simulink model "test_mdl_NI"  (R2018a)
settings: Solver=VariableStepAuto  StartTime=0.0  StopTime=10.0  RelTol=1e-3
(part 23 of 24)

== system test_mdl_NI/CAN_Signal/GWM/Other_GWMTx/CruiseCtrl_Strg_Data_FD1/CcAslButtnSetDecPress2 ==
  in : Inport
  out : Outport
  wires:
  in/1 -> out/1

== system test_mdl_NI/CAN_Signal/GWM/Other_GWMTx/CruiseCtrl_Strg_Data_FD1/CcAslButtnSetIncPress2 ==
  in : Inport
  out : Outport
  wires:
  in/1 -> out/1

== system test_mdl_NI/CAN_Signal/GWM/Other_GWMTx/CruiseCtrl_Strg_Data_FD1/CcAslButtnSetPress2 ==
  in : Inport
  out : Outport
  wires:
  in/1 -> out/1

== system test_mdl_NI/CAN_Signal/GWM/Other_GWMTx/CruiseCtrl_Strg_Data_FD1/CcAsllButtnResPress2 ==
  in : Inport
  out : Outport
  wires:
  in/1 -> out/1

== system test_mdl_NI/CAN_Signal/GWM/Other_GWMTx/CruiseCtrl_Strg_Data_FD1/CcButtnOffPress2 ==
  in : Inport
  out : Outport
  wires:
  in/1 -> out/1

== system test_mdl_NI/CAN_Signal/GWM/Other_GWMTx/CruiseCtrl_Strg_Data_FD1/CcButtnOnOffCnclPress2 ==
  in : Inport
  out : Outport
  wires:
  in/1 -> out/1

== system test_mdl_NI/CAN_Signal/GWM/Other_GWMTx/CruiseCtrl_Strg_Data_FD1/CcButtnOnOffPress2 ==
  in : Inport
  out : Outport
  wires:
  in/1 -> out/1

== system test_mdl_NI/CAN_Signal/GWM/Other_GWMTx/CruiseCtrl_Strg_Data_FD1/CcButtnOnPress2 ==
  in : Inport
  out : Outport
  wires:
  in/1 -> out/1

== system test_mdl_NI/CAN_Signal/GWM/Other_GWMTx/CruiseCtrl_Strg_Data_FD1/SelDrvMdeAdptSte_D_Stat ==
  in : Inport
  out : Outport
  wires:
  in/1 -> out/1

== system test_mdl_NI/CAN_Signal/GWM/Other_GWMTx/CruiseCtrl_Strg_Data_FD1/TjaButtnOnOffPress2 ==
  in : Inport
  out : Outport
  wires:
  in/1 -> out/1

== system test_mdl_NI/CAN_Signal/GWM/Other_GWMTx/DCACA_Data1_FD1/CoolFanDcac_D_Rq ==
  in : Inport
  out : Outport
  wires:
  in/1 -> out/1

== system test_mdl_NI/CAN_Signal/GWM/Other_GWMTx/DCACA_Data1_FD1/DcacClntFlw_D_Rq ==
  in : Inport
  out : Outport
  wires:
  in/1 -> out/1

== system test_mdl_NI/CAN_Signal/GWM/Other_GWMTx/DCACA_Data1_FD1/DcacPlugPrsnt_B_Stat ==
  in : Inport
  out : Outport
  wires:
  in/1 -> out/1

== system test_mdl_NI/CAN_Signal/GWM/Other_GWMTx/DCACA_Data1_FD1/DcacRdy_D_Stat ==
  in : Inport
  out : Outport
  wires:
  in/1 -> out/1

== system test_mdl_NI/CAN_Signal/GWM/Other_GWMTx/DCACA_Data2_FD1/DcacIn_I_Actl ==
  in : Inport
  out : Outport
  wires:
  in/1 -> out/1

== system test_mdl_NI/CAN_Signal/GWM/Other_GWMTx/DCACA_Data2_FD1/DcacIn_U_Actl ==
  in : Inport
  out : Outport
  wires:
  in/1 -> out/1

== system test_mdl_NI/CAN_Signal/GWM/Other_GWMTx/DCACA_Data2_FD1/Dcac_Te_Actl ==
  in : Inport
  out : Outport
  wires:
  in/1 -> out/1

== system test_mdl_NI/CAN_Signal/GWM/Other_GWMTx/DCACA_Data3_FD1/DcacIn_Pw_Mx ==
  in : Inport
  out : Outport
  wires:
  in/1 -> out/1

== system test_mdl_NI/CAN_Signal/GWM/Other_GWMTx/DCACA_Data3_FD1/DcacOut1_Pw_Actl ==
  in : Inport
  out : Outport
  wires:
  in/1 -> out/1

== system test_mdl_NI/CAN_Signal/GWM/Other_GWMTx/DCACA_Data3_FD1/DcacOut2_Pw_Actl ==
  in : Inport
  out : Outport
  wires:
  in/1 -> out/1

== system test_mdl_NI/CAN_Signal/GWM/Other_GWMTx/DCACA_Data3_FD1/DcacOut_Pw_Mx ==
  in : Inport
  out : Outport
  wires:
  in/1 -> out/1

== system test_mdl_NI/CAN_Signal/GWM/Other_GWMTx/DifferentialCtrlData_1_FD1/RearDiffLck_Tq_Actl2 ==
  in : Inport
  out : Outport
  wires:
  in/1 -> out/1

== system test_mdl_NI/CAN_Signal/GWM/Other_GWMTx/Driver_Dr_Stat_FD1/BLISLEDStatDriverSide ==
  in : Inport
  out : Outport
  wires:
  in/1 -> out/1

== system test_mdl_NI/CAN_Signal/GWM/Other_GWMTx/Driver_Dr_Stat_FD1/ChildLckFdbckRd_B_Stat ==
  in : Inport
  out : Outport
  wires:
  in/1 -> out/1

== system test_mdl_NI/CAN_Signal/GWM/Other_GWMTx/Driver_Dr_Stat_FD1/ChildLckPw_D_Rq ==
  in : Inport
  out : Outport
  wires:
  in/1 -> out/1

== system test_mdl_NI/CAN_Signal/GWM/Other_GWMTx/Driver_Dr_Stat_FD1/ChildLckPw_N_Cnt ==
  in : Inport
  out : Outport
  wires:
  in/1 -> out/1

== system test_mdl_NI/CAN_Signal/GWM/Other_GWMTx/Driver_Dr_Stat_FD1/Driver_Lock_Sw_Cnt ==
  in : Inport
  out : Outport
  wires:
  in/1 -> out/1

== system test_mdl_NI/CAN_Signal/GWM/Other_GWMTx/Driver_Dr_Stat_FD1/Driver_Lock_Sw_Stat ==
  in : Inport
  out : Outport
  wires:
  in/1 -> out/1

== system test_mdl_NI/CAN_Signal/GWM/Other_GWMTx/Driver_Dr_Stat_FD1/KeyCylSwDrvDr_D_Stat ==
  in : Inport
  out : Outport
  wires:
  in/1 -> out/1

== system test_mdl_NI/CAN_Signal/GWM/Other_GWMTx/Driver_Dr_Stat_FD1/RollCodeDrvDrKeyCyl ==
  in : Inport
  out : Outport
  wires:
  in/1 -> out/1

== system test_mdl_NI/CAN_Signal/GWM/Other_GWMTx/Driver_Dr_Stat_FD1/RvrseMirrorChime_B_Rq ==
  in : Inport
  out : Outport
  wires:
  in/1 -> out/1

== system test_mdl_NI/CAN_Signal/GWM/Other_GWMTx/Driver_Dr_Stat_FD1/WndwDrvSide_D_Stat ==
  in : Inport
  out : Outport
  wires:
  in/1 -> out/1

== system test_mdl_NI/CAN_Signal/GWM/Other_GWMTx/Dsp_Request_Signals11_FD1/ApaMdeStat_D_RqDrv ==
  in : Inport
  out : Outport
  wires:
  in/1 -> out/1

== system test_mdl_NI/CAN_Signal/GWM/Other_GWMTx/Dsp_Request_Signals11_FD1/ApaSwtch_D_RqMnu ==
  in : Inport
  out : Outport
  wires:
  in/1 -> out/1

== system test_mdl_NI/CAN_Signal/GWM/Other_GWMTx/Dsp_Request_Signals11_FD1/CamAutoTowbarZoom ==
  in : Inport
  out : Outport
  wires:
  in/1 -> out/1

== system test_mdl_NI/CAN_Signal/GWM/Other_GWMTx/Dsp_Request_Signals11_FD1/CamraOvrlDyn_D_Rq ==
  in : Inport
  out : Outport
  wires:
  in/1 -> out/1

== system test_mdl_NI/CAN_Signal/GWM/Other_GWMTx/Dsp_Request_Signals11_FD1/CamraOvrlStat_D_Rq ==
  in : Inport
  out : Outport
  wires:
  in/1 -> out/1

== system test_mdl_NI/CAN_Signal/GWM/Other_GWMTx/Dsp_Request_Signals11_FD1/CamraViewSplit_B_Rq ==
  in : Inport
  out : Outport
  wires:
  in/1 -> out/1

== system test_mdl_NI/CAN_Signal/GWM/Other_GWMTx/Dsp_Request_Signals11_FD1/CamraZoomMan_D_Rq ==
  in : Inport
  out : Outport
  wires:
  in/1 -> out/1

== system test_mdl_NI/CAN_Signal/GWM/Other_GWMTx/Dsp_Request_Signals11_FD1/DistanceBarSetting ==
  in : Inport
  out : Outport
  wires:
  in/1 -> out/1

== system test_mdl_NI/CAN_Signal/GWM/Other_GWMTx/Dsp_Request_Signals11_FD1/PrkAidSwtch_D_RqMnu ==
  in : Inport
  out : Outport
  wires:
  in/1 -> out/1

== system test_mdl_NI/CAN_Signal/GWM/Other_GWMTx/ElecHorizon_Data1_FD1/EhData1_No_Actl ==
  in : Inport
  out : Outport
  wires:
  in/1 -> out/1

== system test_mdl_NI/CAN_Signal/GWM/Other_GWMTx/ElecHorizon_Data2_FD1/EhData2_No_Actl ==
  in : Inport
  out : Outport
  wires:
  in/1 -> out/1

== system test_mdl_NI/CAN_Signal/GWM/Other_GWMTx/FourByFourSwitchData_FD1/AwdLck_D_RqDrv ==
  in : Inport
  out : Outport
  wires:
  in/1 -> out/1

== system test_mdl_NI/CAN_Signal/GWM/Other_GWMTx/FourByFourSwitchData_FD1/AwdMde_D_RqDrv ==
  in : Inport
  out : Outport
  wires:
  in/1 -> out/1

== system test_mdl_NI/CAN_Signal/GWM/Other_GWMTx/FourByFourSwitchData_FD1/DrvSlipCtlMde_B_Rq3 ==
  in : Inport
  out : Outport
  wires:
  in/1 -> out/1

== system test_mdl_NI/CAN_Signal/GWM/Other_GWMTx/FourByFourSwitchData_FD1/HdcSwtchPos_B_Actl ==
  in : Inport
  out : Outport
  wires:
  in/1 -> out/1

== system test_mdl_NI/CAN_Signal/GWM/Other_GWMTx/FourByFourSwitchData_FD1/HybMdeSwtch_B_Rq ==
  in : Inport
  out : Outport
  wires:
  in/1 -> out/1

== system test_mdl_NI/CAN_Signal/GWM/Other_GWMTx/FourByFourSwitchData_FD1/RearDiffLck_D_RqDrv ==
  in : Inport
  out : Outport
  wires:
  in/1 -> out/1

== system test_mdl_NI/CAN_Signal/GWM/Other_GWMTx/FourByFourSwitchData_FD1/TrailCtlSwtch_B_Stat3 ==
  in : Inport
  out : Outport
  wires:
  in/1 -> out/1

== system test_mdl_NI/CAN_Signal/GWM/Other_GWMTx/Front_Distance_Req_FD1/FdsmTrgCntr_B_Actl ==
  in : Inport
  out : Outport
  wires:
  in/1 -> out/1

== system test_mdl_NI/CAN_Signal/GWM/Other_GWMTx/Front_Distance_Req_FD1/FdsmTrgDist_L_Actl ==
  in : Inport
  out : Outport
  wires:
  in/1 -> out/1

== system test_mdl_NI/CAN_Signal/GWM/Other_GWMTx/Front_Distance_Req_FD1/FdsmTrgLeft_B_Actl ==
  in : Inport
  out : Outport
  wires:
  in/1 -> out/1

== system test_mdl_NI/CAN_Signal/GWM/Other_GWMTx/Front_Distance_Req_FD1/FdsmTrgRight_B_Actl ==
  in : Inport
  out : Outport
  wires:
  in/1 -> out/1

== system test_mdl_NI/CAN_Signal/GWM/Other_GWMTx/Front_Distance_Req_FD1/LscmbbBaSens_D_Rq ==
  in : Inport
  out : Outport
  wires:
  in/1 -> out/1

== system test_mdl_NI/CAN_Signal/GWM/Other_GWMTx/Front_Distance_Req_FD1/LscmbbBlck_B_Actl ==
  in : Inport
  out : Outport
  wires:
  in/1 -> out/1

== system test_mdl_NI/CAN_Signal/GWM/Other_GWMTx/Front_Distance_Req_FD1/LscmbbBrkDecel_A_Rq ==
  in : Inport
  out : Outport
  wires:
  in/1 -> out/1

== system test_mdl_NI/CAN_Signal/GWM/Other_GWMTx/Front_Distance_Req_FD1/LscmbbBrkDecel_B_Enbl ==
  in : Inport
  out : Outport
  wires:
  in/1 -> out/1

== system test_mdl_NI/CAN_Signal/GWM/Other_GWMTx/Front_Distance_Req_FD1/LscmbbBrkDecel_No_Cnt ==
  in : Inport
  out : Outport
  wires:
  in/1 -> out/1

== system test_mdl_NI/CAN_Signal/GWM/Other_GWMTx/Front_Distance_Req_FD1/LscmbbBrkDecel_No_Cs ==
  in : Inport
  out : Outport
  wires:
  in/1 -> out/1

== system test_mdl_NI/CAN_Signal/GWM/Other_GWMTx/Front_Distance_Req_FD1/LscmbbBrkPrchg_D_Rq ==
  in : Inport
  out : Outport
  wires:
  in/1 -> out/1

== system test_mdl_NI/CAN_Signal/GWM/Other_GWMTx/Front_Distance_Req_FD1/LscmbbDeny_B_Actl ==
  in : Inport
  out : Outport
  wires:
  in/1 -> out/1

== system test_mdl_NI/CAN_Signal/GWM/Other_GWMTx/Front_Distance_Req_FD1/LscmbbEngTqMn_B_Rq ==
  in : Inport
  out : Outport
  wires:
  in/1 -> out/1

== system test_mdl_NI/CAN_Signal/GWM/Other_GWMTx/Front_Distance_Req_FD1/LscmbbMsgTxt_D_Rq ==
  in : Inport
  out : Outport
  wires:
  in/1 -> out/1

== system test_mdl_NI/CAN_Signal/GWM/Other_GWMTx/Front_Distance_Req_FD1/LscmbbPostEvnt_B_Dsply ==
  in : Inport
  out : Outport
  wires:
  in/1 -> out/1

== system test_mdl_NI/CAN_Signal/GWM/Other_GWMTx/Front_Distance_Req_FD1/LscmbbSrvcRqd_B_Rq ==
  in : Inport
  out : Outport
  wires:
  in/1 -> out/1

== system test_mdl_NI/CAN_Signal/GWM/Other_GWMTx/Front_Distance_Req_FD1/WndwFrontHeat_B_Rq ==
  in : Inport
  out : Outport
  wires:
  in/1 -> out/1

== system test_mdl_NI/CAN_Signal/GWM/Other_GWMTx/GGCC_Config_Mgmt_ID_1_FD1/VehicleGGCCData ==
  in : Inport
  out : Outport
  wires:
  in/1 -> out/1

== system test_mdl_NI/CAN_Signal/GWM/Other_GWMTx/GWM_AutoSar_NetMgmt_FD1/GWM_AutoSarNMControl ==
  in : Inport
  out : Outport
  wires:
  in/1 -> out/1

== system test_mdl_NI/CAN_Signal/GWM/Other_GWMTx/GWM_AutoSar_NetMgmt_FD1/GWM_AutoSarNMNodeId ==
  in : Inport
  out : Outport
  wires:
  in/1 -> out/1

== system test_mdl_NI/CAN_Signal/GWM/Other_GWMTx/GWM_AutoSar_NetMgmt_FD1/GWM_AutoSarNMReserved1 ==
  in : Inport
  out : Outport
  wires:
  in/1 -> out/1

== system test_mdl_NI/CAN_Signal/GWM/Other_GWMTx/GWM_AutoSar_NetMgmt_FD1/GWM_AutoSarNMReserved2 ==
  in : Inport
  out : Outport
  wires:
  in/1 -> out/1

== system test_mdl_NI/CAN_Signal/GWM/Other_GWMTx/GWM_AutoSar_NetMgmt_FD1/GWM_AutoSarNMReserved3 ==
  in : Inport
  out : Outport
  wires:
  in/1 -> out/1

== system test_mdl_NI/CAN_Signal/GWM/Other_GWMTx/GWM_AutoSar_NetMgmt_FD1/GWM_AutoSarNMReserved4 ==
  in : Inport
  out : Outport
  wires:
  in/1 -> out/1

== system test_mdl_NI/CAN_Signal/GWM/Other_GWMTx/GWM_AutoSar_NetMgmt_FD1/GWM_GWNMProxy ==
  in : Inport
  out : Outport
  wires:
  in/1 -> out/1

== system test_mdl_NI/CAN_Signal/GWM/Other_GWMTx/GWM_AutoSar_NetMgmt_FD1/GWM_GWOnBoardTester ==
  in : Inport
  out : Outport
  wires:
  in/1 -> out/1

== system test_mdl_NI/CAN_Signal/GWM/Other_GWMTx/GlobalClock_Data_FD1/GlblClkDay_No_Actl ==
  in : Inport
  out : Outport
  wires:
  in/1 -> out/1

== system test_mdl_NI/CAN_Signal/GWM/Other_GWMTx/GlobalClock_Data_FD1/GlblClkHr_No_Actl ==
  in : Inport
  out : Outport
  wires:
  in/1 -> out/1

== system test_mdl_NI/CAN_Signal/GWM/Other_GWMTx/GlobalClock_Data_FD1/GlblClkMnte_No_Actl ==
  in : Inport
  out : Outport
  wires:
  in/1 -> out/1

== system test_mdl_NI/CAN_Signal/GWM/Other_GWMTx/GlobalClock_Data_FD1/GlblClkScnd_No_Actl ==
  in : Inport
  out : Outport
  wires:
  in/1 -> out/1

== system test_mdl_NI/CAN_Signal/GWM/Other_GWMTx/GlobalClock_Data_FD1/GlblClkYr_No_Actl ==
  in : Inport
  out : Outport
  wires:
  in/1 -> out/1

== system test_mdl_NI/CAN_Signal/GWM/Other_GWMTx/Global_PATS_Cntrl_Info_FD1/immoControlCmd_T1 ==
  in : Inport
  out : Outport
  wires:
  in/1 -> out/1

== system test_mdl_NI/CAN_Signal/GWM/Other_GWMTx/Global_PATS_Cntrl_Info_FD1/immoControlData_T1 ==
  in : Inport
  out : Outport
  wires:
  in/1 -> out/1

== system test_mdl_NI/CAN_Signal/GWM/Other_GWMTx/IPC_Infotainment_FD1/BeltminderAudioMute ==
  in : Inport
  out : Outport
  wires:
  in/1 -> out/1

== system test_mdl_NI/CAN_Signal/GWM/Other_GWMTx/IPC_Infotainment_FD1/Chime_Source ==
  in : Inport
  out : Outport
  wires:
  in/1 -> out/1

== system test_mdl_NI/CAN_Signal/GWM/Other_GWMTx/IPC_Infotainment_FD1/HdcOn_B_Rq ==
  in : Inport
  out : Outport
  wires:
  in/1 -> out/1

== system test_mdl_NI/CAN_Signal/GWM/Other_GWMTx/IPC_Infotainment_FD1/IPC_Attn_Info_Audio ==
  in : Inport
  out : Outport
  wires:
  in/1 -> out/1

== system test_mdl_NI/CAN_Signal/GWM/Other_GWMTx/IPC_Infotainment_FD1/IPC_MyKeyVolLimit_St ==
  in : Inport
  out : Outport
  wires:
  in/1 -> out/1

== system test_mdl_NI/CAN_Signal/GWM/Other_GWMTx/IPC_Infotainment_FD1/IPC_New_Attn_Event ==
  in : Inport
  out : Outport
  wires:
  in/1 -> out/1

== system test_mdl_NI/CAN_Signal/GWM/Other_GWMTx/IPC_Infotainment_FD1/Power_Up_Chime_Modules ==
  in : Inport
  out : Outport
  wires:
  in/1 -> out/1

== system test_mdl_NI/CAN_Signal/GWM/Other_GWMTx/IPC_Infotainment_FD1/Veh_V2_Dsply ==
  in : Inport
  out : Outport
  wires:
  in/1 -> out/1

== system test_mdl_NI/CAN_Signal/GWM/Other_GWMTx/IPC_Send_Signals_2_FD1/ElLongTerm_L_Dsply ==
  in : Inport
  out : Outport
  wires:
  in/1 -> out/1

== system test_mdl_NI/CAN_Signal/GWM/Other_GWMTx/IPC_Send_Signals_2_FD1/ElTrip_L_Dsply ==
  in : Inport
  out : Outport
  wires:
  in/1 -> out/1

== system test_mdl_NI/CAN_Signal/GWM/Other_GWMTx/IPC_Send_Signals_2_FD1/FuelRange_L_Dsply ==
  in : Inport
  out : Outport
  wires:
  in/1 -> out/1

== system test_mdl_NI/CAN_Signal/GWM/Other_GWMTx/MHT_EV_Wakeup_FD1/BattChlrSov_B_Rq ==
  in : Inport
  out : Outport
  wires:
  in/1 -> out/1

== system test_mdl_NI/CAN_Signal/GWM/Other_GWMTx/MHT_EV_Wakeup_FD1/BattChrgTrgtSoC_D_Rq ==
  in : Inport
  out : Outport
  wires:
  in/1 -> out/1

== system test_mdl_NI/CAN_Signal/GWM/Other_GWMTx/MHT_EV_Wakeup_FD1/BattTracDrvSustn_B_Rq ==
  in : Inport
  out : Outport
  wires:
  in/1 -> out/1

== system test_mdl_NI/CAN_Signal/GWM/Other_GWMTx/MHT_EV_Wakeup_FD1/BrkAppl_D_RqPt ==
  in : Inport
  out : Outport
  wires:
  in/1 -> out/1

== system test_mdl_NI/CAN_Signal/GWM/Other_GWMTx/MHT_EV_Wakeup_FD1/CabnEvapSovFront_B_Rq ==
  in : Inport
  out : Outport
  wires:
  in/1 -> out/1

== system test_mdl_NI/CAN_Signal/GWM/Other_GWMTx/MHT_EV_Wakeup_FD1/CabnEvapSovRear_B_Rq ==
  in : Inport
  out : Outport
  wires:
  in/1 -> out/1

== system test_mdl_NI/CAN_Signal/GWM/Other_GWMTx/MHT_EV_Wakeup_FD1/HeatCoreSovRear_B_Rq ==
  in : Inport
  out : Outport
  wires:
  in/1 -> out/1

== system test_mdl_NI/CAN_Signal/GWM/Other_GWMTx/MHT_EV_Wakeup_FD1/HtrnClntFlw_D_Rq ==
  in : Inport
  out : Outport
  wires:
  in/1 -> out/1

== system test_mdl_NI/CAN_Signal/GWM/Other_GWMTx/MHT_EV_Wakeup_FD1/HtrnCnnctPwr_B_Stat ==
  in : Inport
  out : Outport
  wires:
  in/1 -> out/1

== system test_mdl_NI/CAN_Signal/GWM/Other_GWMTx/MHT_EV_Wakeup_FD1/HtrnDcdcDis_B_Rq ==
  in : Inport
  out : Outport
  wires:
  in/1 -> out/1

== system test_mdl_NI/CAN_Signal/GWM/Other_GWMTx/MHT_EV_Wakeup_FD1/PtcHtr_D_Stat ==
  in : Inport
  out : Outport
  wires:
  in/1 -> out/1

== system test_mdl_NI/CAN_Signal/GWM/Other_GWMTx/Mc_Send_Signals_2_FD1/BttOn_B_Rq ==
  in : Inport
  out : Outport
  wires:
  in/1 -> out/1

== system test_mdl_NI/CAN_Signal/GWM/Other_GWMTx/Mc_Send_Signals_2_FD1/Btt_L_Actl ==
  in : Inport
  out : Outport
  wires:
  in/1 -> out/1

== system test_mdl_NI/CAN_Signal/GWM/Other_GWMTx/Mc_Send_Signals_2_FD1/EngExhMdeQuiet_D_Rq ==
  in : Inport
  out : Outport
  wires:
  in/1 -> out/1

== system test_mdl_NI/CAN_Signal/GWM/Other_GWMTx/Mc_Send_Signals_2_FD1/EsaOn_B_Rq ==
  in : Inport
  out : Outport
  wires:
  in/1 -> out/1

== system test_mdl_NI/CAN_Signal/GWM/Other_GWMTx/Mc_Send_Signals_2_FD1/Mc_VehLangUsrSel_St ==
  in : Inport
  out : Outport
  wires:
  in/1 -> out/1

== system test_mdl_NI/CAN_Signal/GWM/Other_GWMTx/Mc_Send_Signals_2_FD1/Mc_VehUnitTempUsrSel_St ==
  in : Inport
  out : Outport
  wires:
  in/1 -> out/1

== system test_mdl_NI/CAN_Signal/GWM/Other_GWMTx/Mc_Send_Signals_2_FD1/Mc_VehUntTrpCoUsrSel_St ==
  in : Inport
  out : Outport
  wires:
  in/1 -> out/1

== system test_mdl_NI/CAN_Signal/GWM/Other_GWMTx/Mc_Send_Signals_2_FD1/SelDrvMdeDsply_B_Avail ==
  in : Inport
  out : Outport
  wires:
  in/1 -> out/1

== system test_mdl_NI/CAN_Signal/GWM/Other_GWMTx/Mc_Send_Signals_2_FD1/SelDrvMdeTxtReset_B_Rq ==
  in : Inport
  out : Outport
  wires:
  in/1 -> out/1

== system test_mdl_NI/CAN_Signal/GWM/Other_GWMTx/Mc_Send_Signals_2_FD1/WaitToStartLamp_D_Falt ==
  in : Inport
  out : Outport
  wires:
  in/1 -> out/1

== system test_mdl_NI/CAN_Signal/GWM/Other_GWMTx/ParkAid_Aud_Warn_CmdM_FD1/Cta_D_Rq ==
  in : Inport
  out : Outport
  wires:
  in/1 -> out/1

== system test_mdl_NI/CAN_Signal/GWM/Other_GWMTx/ParkAid_Aud_Warn_CmdM_FD1/PrkAidRear_D_RqDrv ==
  in : Inport
  out : Outport
  wires:
  in/1 -> out/1

== system test_mdl_NI/CAN_Signal/GWM/Other_GWMTx/ParkAid_Aud_Warn_CmdM_FD1/Sod_D_Rq ==
  in : Inport
  out : Outport
  wires:
  in/1 -> out/1

== system test_mdl_NI/CAN_Signal/GWM/Other_GWMTx/ParkAid_Aud_Warn_CmdM_FD1/SteEffort_D_Rq ==
  in : Inport
  out : Outport
  wires:
  in/1 -> out/1

== system test_mdl_NI/CAN_Signal/GWM/Other_GWMTx/Pass_Dr_Stat_FD1/BLISLEDStatPassSide ==
  in : Inport
  out : Outport
  wires:
  in/1 -> out/1

== system test_mdl_NI/CAN_Signal/GWM/Other_GWMTx/Pass_Dr_Stat_FD1/ChildLckFdbckRp_B_Stat ==
  in : Inport
  out : Outport
  wires:
  in/1 -> out/1

== system test_mdl_NI/CAN_Signal/GWM/Other_GWMTx/Pass_Dr_Stat_FD1/Memory_1_SwPsngr_Stat ==
  in : Inport
  out : Outport
  wires:
  in/1 -> out/1

== system test_mdl_NI/CAN_Signal/GWM/Other_GWMTx/Pass_Dr_Stat_FD1/Memory_2_SwPsngr_Stat ==
  in : Inport
  out : Outport
  wires:
  in/1 -> out/1

== system test_mdl_NI/CAN_Signal/GWM/Other_GWMTx/Pass_Dr_Stat_FD1/Memory_3_SwPsngr_Stat ==
  in : Inport
  out : Outport
  wires:
  in/1 -> out/1

== system test_mdl_NI/CAN_Signal/GWM/Other_GWMTx/Pass_Dr_Stat_FD1/Pasngr_Lock_Sw_Cnt ==
  in : Inport
  out : Outport
  wires:
  in/1 -> out/1

== system test_mdl_NI/CAN_Signal/GWM/Other_GWMTx/Pass_Dr_Stat_FD1/Pasngr_Lock_Sw_Stat ==
  in : Inport
  out : Outport
  wires:
  in/1 -> out/1

== system test_mdl_NI/CAN_Signal/GWM/Other_GWMTx/Pass_Dr_Stat_FD1/RollCode_No_ActlPdm ==
  in : Inport
  out : Outport
  wires:
  in/1 -> out/1

== system test_mdl_NI/CAN_Signal/GWM/Other_GWMTx/Pass_Dr_Stat_FD1/WndwPsngrSide_D_Stat ==
  in : Inport
  out : Outport
  wires:
  in/1 -> out/1

== system test_mdl_NI/CAN_Signal/GWM/Other_GWMTx/Personality_APIM_Data_FD1/CtrStkDsplyOp_D_Rq ==
  in : Inport
  out : Outport
  wires:
  in/1 -> out/1

== system test_mdl_NI/CAN_Signal/GWM/Other_GWMTx/Personality_APIM_Data_FD1/CtrStkFeatConfigActl ==
  in : Inport
  out : Outport
  wires:
  in/1 -> out/1

== system test_mdl_NI/CAN_Signal/GWM/Other_GWMTx/Personality_APIM_Data_FD1/CtrStkFeatNoActl ==
  in : Inport
  out : Outport
  wires:
  in/1 -> out/1

== system test_mdl_NI/CAN_Signal/GWM/Other_GWMTx/Personality_APIM_Data_FD1/CtrStkPersIndex_D_Actl ==
  in : Inport
  out : Outport
  wires:
  in/1 -> out/1

== system test_mdl_NI/CAN_Signal/GWM/Other_GWMTx/Personality_APIM_Data_FD1/Pers1OptIn_B_Stats ==
  in : Inport
  out : Outport
  wires:
  in/1 -> out/1

== system test_mdl_NI/CAN_Signal/GWM/Other_GWMTx/Personality_APIM_Data_FD1/Pers2OptIn_B_Stats ==
  in : Inport
  out : Outport
  wires:
  in/1 -> out/1

== system test_mdl_NI/CAN_Signal/GWM/Other_GWMTx/Personality_APIM_Data_FD1/Pers3OptIn_B_Stats ==
  in : Inport
  out : Outport
  wires:
  in/1 -> out/1

== system test_mdl_NI/CAN_Signal/GWM/Other_GWMTx/Personality_APIM_Data_FD1/Pers4OptIn_B_Stats ==
  in : Inport
  out : Outport
  wires:
  in/1 -> out/1

== system test_mdl_NI/CAN_Signal/GWM/Other_GWMTx/Personality_APIM_Data_FD1/PersStore_D_Rq ==
  in : Inport
  out : Outport
  wires:
  in/1 -> out/1

== system test_mdl_NI/CAN_Signal/GWM/Other_GWMTx/Personality_Data_FD1/MsgCntrDsplyOp_D_Rq ==
  in : Inport
  out : Outport
  wires:
  in/1 -> out/1

== system test_mdl_NI/CAN_Signal/GWM/Other_GWMTx/Personality_Data_FD1/MsgCntrFeatConfigRq ==
  in : Inport
  out : Outport
  wires:
  in/1 -> out/1

== system test_mdl_NI/CAN_Signal/GWM/Other_GWMTx/Personality_Data_FD1/MsgCntrFeatNoRq ==
  in : Inport
  out : Outport
  wires:
  in/1 -> out/1

== system test_mdl_NI/CAN_Signal/GWM/Other_GWMTx/Personality_Data_FD1/MsgCntrPersIndex_D_Rq ==
  in : Inport
  out : Outport
  wires:
  in/1 -> out/1

== system test_mdl_NI/CAN_Signal/GWM/Other_GWMTx/Power_Liftgate_Stat_FD1/DrLckCnt_No_ActlTgate ==
  in : Inport
  out : Outport
  wires:
  in/1 -> out/1

== system test_mdl_NI/CAN_Signal/GWM/Other_GWMTx/Power_Liftgate_Stat_FD1/DrTGate_D_Rq ==
  in : Inport
  out : Outport
  wires:
  in/1 -> out/1

== system test_mdl_NI/CAN_Signal/GWM/Other_GWMTx/Power_Liftgate_Stat_FD1/DrTgateChime2_D_Rq ==
  in : Inport
  out : Outport
  wires:
  in/1 -> out/1

== system test_mdl_NI/CAN_Signal/GWM/Other_GWMTx/Power_Liftgate_Stat_FD1/Power_Liftgate_Mode_Stt ==
  in : Inport
  out : Outport
  wires:
  in/1 -> out/1

== system test_mdl_NI/CAN_Signal/GWM/Other_GWMTx/Power_Liftgate_Stat_FD1/PwLftgtIntSw_B_Stat ==
  in : Inport
  out : Outport
  wires:
  in/1 -> out/1

== system test_mdl_NI/CAN_Signal/GWM/Other_GWMTx/PreCond_Hev_Data1_FD1/ChrgStat_D2_Dsply ==
  in : Inport
  out : Outport
  wires:
  in/1 -> out/1

== system test_mdl_NI/CAN_Signal/GWM/Other_GWMTx/PreCond_Hev_Data2_FD1/BattTracClntFlw_Pc_Rq ==
  in : Inport
  out : Outport
  wires:
  in/1 -> out/1

== system test_mdl_NI/CAN_Signal/GWM/Other_GWMTx/PreCond_Hev_Data2_FD1/BattTrac_I_EstVsc ==
  in : Inport
  out : Outport
  wires:
  in/1 -> out/1

== system test_mdl_NI/CAN_Signal/GWM/Other_GWMTx/PreCond_Hev_Data2_FD1/DrvCondTpRrDefrs_B_Rq ==
  in : Inport
  out : Outport
  wires:
  in/1 -> out/1

== system test_mdl_NI/CAN_Signal/GWM/Other_GWMTx/PreCond_Hev_Data2_FD1/HtrnAin_UHi_Actl ==
  in : Inport
  out : Outport
  wires:
  in/1 -> out/1

== system test_mdl_NI/CAN_Signal/GWM/Other_GWMTx/PreCond_Hev_Data2_FD1/HtrnHvilOpen_B_Actl ==
  in : Inport
  out : Outport
  wires:
  in/1 -> out/1

== system test_mdl_NI/CAN_Signal/GWM/Other_GWMTx/PreCond_Hev_Data2_FD1/HtrnMil_D_Rq ==
  in : Inport
  out : Outport
  wires:
  in/1 -> out/1

== system test_mdl_NI/CAN_Signal/GWM/Other_GWMTx/PreCond_Hev_Data2_FD1/HtrnOvrTeLamp_B_Dsply ==
  in : Inport
  out : Outport
  wires:
  in/1 -> out/1

== system test_mdl_NI/CAN_Signal/GWM/Other_GWMTx/PreCond_Hev_Data2_FD1/HtrnSrvcRqd_B_Dsply ==
  in : Inport
  out : Outport
  wires:
  in/1 -> out/1

== system test_mdl_NI/CAN_Signal/GWM/Other_GWMTx/PreCond_Hev_Data2_FD1/PreCondActv_B_Actl ==
  in : Inport
  out : Outport
  wires:
  in/1 -> out/1

== system test_mdl_NI/CAN_Signal/GWM/Other_GWMTx/PreCond_Hev_Data2_FD1/PtWakeupDeltaT_T_Rq ==
  in : Inport
  out : Outport
  wires:
  in/1 -> out/1

== system test_mdl_NI/CAN_Signal/GWM/Other_GWMTx/Suspension_Data_FD1/SuspClkSync_No_Rq ==
  in : Inport
  out : Outport
  wires:
  in/1 -> out/1

== system test_mdl_NI/CAN_Signal/GWM/Other_GWMTx/Suspension_Data_FD1/SuspFrntRight_L_Actl ==
  in : Inport
  out : Outport
  wires:
  in/1 -> out/1

== system test_mdl_NI/CAN_Signal/GWM/Other_GWMTx/Suspension_Data_FD1/SuspFrnt_L_Actl ==
  in : Inport
  out : Outport
  wires:
  in/1 -> out/1

== system test_mdl_NI/CAN_Signal/GWM/Other_GWMTx/Suspension_Data_FD1/SuspFrnt_L_Prev ==
  in : Inport
  out : Outport
  wires:
  in/1 -> out/1

== system test_mdl_NI/CAN_Signal/GWM/Other_GWMTx/Suspension_Data_FD1/SuspRearRight_L_Actl ==
  in : Inport
  out : Outport
  wires:
  in/1 -> out/1

== system test_mdl_NI/CAN_Signal/GWM/Other_GWMTx/Suspension_Data_FD1/SuspRear_L_Actl ==
  in : Inport
  out : Outport
  wires:
  in/1 -> out/1

== system test_mdl_NI/CAN_Signal/GWM/Other_GWMTx/Suspension_Data_FD1/SuspRear_L_Prev ==
  in : Inport
  out : Outport
  wires:
  in/1 -> out/1

== system test_mdl_NI/CAN_Signal/GWM/Other_GWMTx/TesterPhysicalResGWM_FD1/TesterPhysicalResGWM_F1 ==
  in : Inport
  out : Outport
  wires:
  in/1 -> out/1

== system test_mdl_NI/CAN_Signal/GWM/Other_GWMTx/TrailerAid_Data_FD1/TrlBrkInitOut_D_Rq ==
  in : Inport
  out : Outport
  wires:
  in/1 -> out/1

== system test_mdl_NI/CAN_Signal/GWM/Other_GWMTx/TrailerAid_Data_FD1/TrlrAidEnbl_D_Rq ==
  in : Inport
  out : Outport
  wires:
  in/1 -> out/1

== system test_mdl_NI/CAN_Signal/GWM/Other_GWMTx/TrailerAid_Data_FD1/TrlrAidSetup_D_Rq ==
  in : Inport
  out : Outport
  wires:
  in/1 -> out/1

== system test_mdl_NI/CAN_Signal/GWM/Other_GWMTx/TrailerAid_Data_FD1/TrlrAnOffstDir_D_Mem ==
  in : Inport
  out : Outport
  wires:
  in/1 -> out/1

== system test_mdl_NI/CAN_Signal/GWM/Other_GWMTx/TrailerAid_Data_FD1/TrlrAnOffst_An_Mem ==
  in : Inport
  out : Outport
  wires:
  in/1 -> out/1

== system test_mdl_NI/CAN_Signal/GWM/Other_GWMTx/TrailerAid_Data_FD1/TrlrAxleToBmpr_L_Actl ==
  in : Inport
  out : Outport
  wires:
  in/1 -> out/1

== system test_mdl_NI/CAN_Signal/GWM/Other_GWMTx/TrailerAid_Data_FD1/TrlrBallToBmpr_L_Actl ==
  in : Inport
  out : Outport
  wires:
  in/1 -> out/1

== system test_mdl_NI/CAN_Signal/GWM/Other_GWMTx/TrailerAid_Data_FD1/TrlrId_No_Actl ==
  in : Inport
  out : Outport
  wires:
  in/1 -> out/1

== system test_mdl_NI/CAN_Signal/GWM/Other_GWMTx/TrailerAid_Data_FD1/TrlrRvrseCancl_B_Rq ==
  in : Inport
  out : Outport
  wires:
  in/1 -> out/1

== system test_mdl_NI/CAN_Signal/GWM/Other_GWMTx/TrailerAid_Data_FD1/TrlrTrgtOffst_L_Actl ==
  in : Inport
  out : Outport
  wires:
  in/1 -> out/1

== system test_mdl_NI/CAN_Signal/GWM/Other_GWMTx/TrailerAid_Data_FD1/TrlrTrgtPtrnId_No_Mem ==
  in : Inport
  out : Outport
  wires:
  in/1 -> out/1

== system test_mdl_NI/CAN_Signal/GWM/Other_GWMTx/TrailerAid_Data_FD1/TrlrTrgtToBmpr_L_Actl ==
  in : Inport
  out : Outport
  wires:
  in/1 -> out/1

== system test_mdl_NI/CAN_Signal/GWM/Other_GWMTx/TrailerAid_Stat1_FD1/TrlrSnsId_No_Actl ==
  in : Inport
  out : Outport
  wires:
  in/1 -> out/1

== system test_mdl_NI/CAN_Signal/GWM/Other_GWMTx/TrailerAid_Stat2_FD1/TrlrHitYaw_AnRate_Actl ==
  in : Inport
  out : Outport
  wires:
  in/1 -> out/1

== system test_mdl_NI/CAN_Signal/GWM/Other_GWMTx/TrailerAid_Stat2_FD1/TrlrHitchYaw_An_Actl ==
  in : Inport
  out : Outport
  wires:
  in/1 -> out/1

== system test_mdl_NI/CAN_Signal/GWM/Other_GWMTx/TrailerAid_Stat2_FD1/TrlrHitchYaw_D_Stat ==
  in : Inport
  out : Outport
  wires:
  in/1 -> out/1

== system test_mdl_NI/CAN_Signal/GWM/Other_GWMTx/TrailerAid_Stat2_FD1/TrlrYawWActl_D_Qf ==
  in : Inport
  out : Outport
  wires:
  in/1 -> out/1

== system test_mdl_NI/CAN_Signal/GWM/Other_GWMTx/TrailerAid_Stat2_FD1/TrlrYaw_W_Actl ==
  in : Inport
  out : Outport
  wires:
  in/1 -> out/1

== system test_mdl_NI/CAN_Signal/GWM/Other_GWMTx/TrailerBrakeInfo_FD1/StopLamp_B_RqTrlrBrk ==
  in : Inport
  out : Outport
  wires:
  in/1 -> out/1

== system test_mdl_NI/CAN_Signal/GWM/Other_GWMTx/TrailerBrakeInfo_FD1/TrlBrkInitOut_D_Stat ==
  in : Inport
  out : Outport
  wires:
  in/1 -> out/1

== system test_mdl_NI/CAN_Signal/GWM/Other_GWMTx/TrailerBrakeInfo_FD1/TrlrBrkActCirct_B_Falt ==
  in : Inport
  out : Outport
  wires:
  in/1 -> out/1

== system test_mdl_NI/CAN_Signal/GWM/Other_GWMTx/TrailerBrakeInfo_FD1/TrlrBrkActCnnct_B_Actl ==
  in : Inport
  out : Outport
  wires:
  in/1 -> out/1

== system test_mdl_NI/CAN_Signal/GWM/Other_GWMTx/TrailerBrakeInfo_FD1/TrlrBrkCtl_B_Falt ==
  in : Inport
  out : Outport
  wires:
  in/1 -> out/1

== system test_mdl_NI/CAN_Signal/GWM/Other_GWMTx/TrailerBrakeInfo_FD1/TrlrBrkDcnnt_B_Actl ==
  in : Inport
  out : Outport
  wires:
  in/1 -> out/1

== system test_mdl_NI/CAN_Signal/GWM/Other_GWMTx/TrailerBrakeInfo_FD1/TrlrBrkDsply_B_Rq ==
  in : Inport
  out : Outport
  wires:
  in/1 -> out/1

== system test_mdl_NI/CAN_Signal/GWM/Other_GWMTx/TrailerBrakeInfo_FD1/TrlrBrkGain_No_Actl ==
  in : Inport
  out : Outport
  wires:
  in/1 -> out/1

== system test_mdl_NI/CAN_Signal/GWM/Other_GWMTx/TrailerBrakeInfo_FD1/TrlrBrkMde_D_Actl ==
  in : Inport
  out : Outport
  wires:
  in/1 -> out/1

== system test_mdl_NI/CAN_Signal/GWM/Other_GWMTx/TrailerBrakeInfo_FD1/TrlrBrkOut_No_Dsply ==
  in : Inport
  out : Outport
  wires:
  in/1 -> out/1

== system test_mdl_NI/CAN_Signal/GWM/Other_GWMTx/TrailerInfo_2_FD1/TrlrAidAn_URate_Actl ==
  in : Inport
  out : Outport
  wires:
  in/1 -> out/1

== system test_mdl_NI/CAN_Signal/GWM/Other_GWMTx/TrailerInfo_2_FD1/TrlrAidAn_U_Actl ==
  in : Inport
  out : Outport
  wires:
  in/1 -> out/1

== system test_mdl_NI/CAN_Signal/GWM/Other_GWMTx/TrailerInfo_2_FD1/TrlrAidCtl_U_RqDrv ==
  in : Inport
  out : Outport
  wires:
  in/1 -> out/1

== system test_mdl_NI/CAN_Signal/GWM/Other_GWMTx/TrailerInfo_2_FD1/TrlrAidSwtch_D_RqDrv ==
  in : Inport
  out : Outport
  wires:
  in/1 -> out/1

== system test_mdl_NI/CAN_Signal/GWM/Other_GWMTx/TrailerInfo_FD1/ParkLampTrlrOut_B_Stat ==
  in : Inport
  out : Outport
  wires:
  in/1 -> out/1

== system test_mdl_NI/CAN_Signal/GWM/Other_GWMTx/TrailerInfo_FD1/StopLampTrlrOut_B_Stat ==
  in : Inport
  out : Outport
  wires:
  in/1 -> out/1

== system test_mdl_NI/CAN_Signal/GWM/Other_GWMTx/TrailerInfo_FD1/TrlrBattChrg_D_Stat ==
  in : Inport
  out : Outport
  wires:
  in/1 -> out/1

== system test_mdl_NI/CAN_Signal/GWM/Other_GWMTx/TrailerInfo_FD1/TrlrLampCnnct_B_Actl ==
  in : Inport
  out : Outport
  wires:
  in/1 -> out/1

== system test_mdl_NI/CAN_Signal/GWM/Other_GWMTx/TrailerInfo_FD1/TrlrLampCtl_D_Stat ==
  in : Inport
  out : Outport
  wires:
  in/1 -> out/1

== system test_mdl_NI/CAN_Signal/GWM/Other_GWMTx/TrailerInfo_FD1/TurnLampTrlrRl_B_Stat ==
  in : Inport
  out : Outport
  wires:
  in/1 -> out/1

== system test_mdl_NI/CAN_Signal/GWM/Other_GWMTx/TrailerInfo_FD1/TurnLampTrlrRr_B_Stat ==
  in : Inport
  out : Outport
  wires:
  in/1 -> out/1

== system test_mdl_NI/CAN_Signal/GWM/Other_GWMTx/VeyDynamics_Data_FD1/AdptDrvMdeChassis_D_Rq ==
  in : Inport
  out : Outport
  wires:
  in/1 -> out/1

== system test_mdl_NI/CAN_Signal/GWM/Other_GWMTx/VeyDynamics_Data_FD1/AdptDrvMdePt_D_Rq ==
  in : Inport
  out : Outport
  wires:
  in/1 -> out/1

== system test_mdl_NI/CAN_Signal/GWM/Other_GWMTx/VeyDynamics_Data_FD1/AirSprngRateFl_D_Rq ==
  in : Inport
  out : Outport
  wires:
  in/1 -> out/1

== system test_mdl_NI/CAN_Signal/GWM/Other_GWMTx/VeyDynamics_Data_FD1/AirSprngRateFr_D_Rq ==
  in : Inport
  out : Outport
  wires:
  in/1 -> out/1

== system test_mdl_NI/CAN_Signal/GWM/Other_GWMTx/VeyDynamics_Data_FD1/AirSprngRateRl_D_Rq ==
  in : Inport
  out : Outport
  wires:
  in/1 -> out/1

== system test_mdl_NI/CAN_Signal/GWM/Other_GWMTx/VeyDynamics_Data_FD1/AirSprngRateRr_D_Rq ==
  in : Inport
  out : Outport
  wires:
  in/1 -> out/1

== system test_mdl_NI/CAN_Signal/GWM/Other_GWMTx/VeyDynamics_Data_FD1/AirSuspMsgTxt_D_Rq ==
  in : Inport
  out : Outport
  wires:
  in/1 -> out/1

== system test_mdl_NI/CAN_Signal/GWM/Other_GWMTx/VeyDynamics_Data_FD1/AirSusp_D_Stat ==
  in : Inport
  out : Outport
  wires:
  in/1 -> out/1

== system test_mdl_NI/CAN_Signal/GWM/Other_GWMTx/VeyDynamics_Data_FD1/BrkPadMsgTxt_D_Rq ==
  in : Inport
  out : Outport
  wires:
  in/1 -> out/1

== system test_mdl_NI/CAN_Signal/GWM/Other_GWMTx/VeyDynamics_Data_FD1/CcdMsgTxt_D_RqDsply ==
  in : Inport
  out : Outport
  wires:
  in/1 -> out/1

== system test_mdl_NI/CAN_Signal/GWM/Other_GWMTx/VeyDynamics_Data_FD1/Ccd_B_Falt ==
  in : Inport
  out : Outport
  wires:
  in/1 -> out/1

== system test_mdl_NI/CAN_Signal/GWM/Other_GWMTx/VeyDynamics_Data_FD1/SelDrvMdeSusp_D_Stat ==
  in : Inport
  out : Outport
  wires:
  in/1 -> out/1

== system test_mdl_NI/CAN_Signal/GWM/Other_GWMTx/VeyDynamics_Data_FD1/SuspDrvMde_D_Stat ==
  in : Inport
  out : Outport
  wires:
  in/1 -> out/1

== system test_mdl_NI/CAN_Signal/GWM/Other_GWMTx/VeyDynamics_Data_FD1/SuspType_B_Stat ==
  in : Inport
  out : Outport
  wires:
  in/1 -> out/1

== system test_mdl_NI/CAN_Signal/GWM/Other_GWMTx/VeyDynamics_Data_FD1/SuspVLim_B_Rq ==
  in : Inport
  out : Outport
  wires:
  in/1 -> out/1

== system test_mdl_NI/CAN_Signal/GWM/RCM/RCMSerialNumber_FD1_454/RCMSerialNoByte1 ==
  in : Inport
  out : Outport
  wires:
  in/1 -> out/1

== system test_mdl_NI/CAN_Signal/GWM/RCM/RCMSerialNumber_FD1_454/RCMSerialNoByte2 ==
  in : Inport
  out : Outport
  wires:
  in/1 -> out/1

== system test_mdl_NI/CAN_Signal/GWM/RCM/RCMSerialNumber_FD1_454/RCMSerialNoByte3 ==
  in : Inport
  out : Outport
  wires:
  in/1 -> out/1

== system test_mdl_NI/CAN_Signal/GWM/RCM/RCMSerialNumber_FD1_454/RCMSerialNoByte4 ==
  in : Inport
  out : Outport
  wires:
  in/1 -> out/1

== system test_mdl_NI/CAN_Signal/GWM/RCM/RCMSerialNumber_FD1_454/RCMSerialNoByte5 ==
  in : Inport
  out : Outport
  wires:
  in/1 -> out/1

== system test_mdl_NI/CAN_Signal/GWM/RCM/RCMSerialNumber_FD1_454/RCMSerialNoByte6 ==
  in : Inport
  out : Outport
  wires:
  in/1 -> out/1

== system test_mdl_NI/CAN_Signal/GWM/RCM/RCMSerialNumber_FD1_454/RCMSerialNoByte7 ==
  in : Inport
  out : Outport
  wires:
  in/1 -> out/1

== system test_mdl_NI/CAN_Signal/GWM/RCM/RCMSerialNumber_FD1_454/RCMSerialNoByte8 ==
  in : Inport
  out : Outport
  wires:
  in/1 -> out/1

== system test_mdl_NI/CAN_Signal/GWM/RCM/RCMStatusMessage2_FD1_4C/EDRTriggerEvntSync ==
  in : Inport
  out : Outport
  wires:
  in/1 -> out/1

== system test_mdl_NI/CAN_Signal/GWM/RCM/RCMStatusMessage2_FD1_4C/FirstRowBuckleDriver ==
  in : Inport
  out : Outport
  wires:
  in/1 -> out/1

== system test_mdl_NI/CAN_Signal/GWM/RCM/RCMStatusMessage2_FD1_4C/FirstRowBuckleMid ==
  in : Inport
  out : Outport
  wires:
  in/1 -> out/1

== system test_mdl_NI/CAN_Signal/GWM/RCM/RCMStatusMessage2_FD1_4C/FirstRowBucklePsngr ==
  in : Inport
  out : Outport
  wires:
  in/1 -> out/1

== system test_mdl_NI/CAN_Signal/GWM/RCM/RCMStatusMessage2_FD1_4C/PassRstrnInd_Req ==
  in : Inport
  out : Outport
  wires:
  in/1 -> out/1

== system test_mdl_NI/CAN_Signal/GWM/RCM/RCMStatusMessage2_FD1_4C/PsngrFmidDetct_D_Actl ==
  in : Inport
  out : Outport
  wires:
  in/1 -> out/1

== system test_mdl_NI/CAN_Signal/GWM/RCM/RCMStatusMessage2_FD1_4C/PsngrFrntDetct_D_Actl ==
  in : Inport
  out : Outport
  wires:
  in/1 -> out/1

== system test_mdl_NI/CAN_Signal/GWM/RCM/RCMStatusMessage2_FD1_4C/RILReq ==
  in : Inport
  out : Outport
  wires:
  in/1 -> out/1

== system test_mdl_NI/CAN_Signal/GWM/RCM/RCMStatusMessage2_FD1_4C/RstrnImpactEvntStatus ==
  in : Inport
  out : Outport
  wires:
  in/1 -> out/1

== system test_mdl_NI/CAN_Signal/GWM/RCM/RCMStatusMessage2_FD1_4C/RstrnPsngrOn_D_Stat ==
  in : Inport
  out : Outport
  wires:
  in/1 -> out/1

== system test_mdl_NI/CAN_Signal/GWM/RCM/RCMStatusMessage2_FD1_4C/SecondRowBuckleDriver ==
  in : Inport
  out : Outport
  wires:
  in/1 -> out/1

== system test_mdl_NI/CAN_Signal/GWM/RCM/RCMStatusMessage2_FD1_4C/SecondRowBuckleMid ==
  in : Inport
  out : Outport
  wires:
  in/1 -> out/1

== system test_mdl_NI/CAN_Signal/GWM/RCM/RCMStatusMessage2_FD1_4C/SecondRowBucklePsngr ==
  in : Inport
  out : Outport
  wires:
  in/1 -> out/1

== system test_mdl_NI/CAN_Signal/GWM/RCM/RCMStatusMessage2_FD1_4C/ThirdRowBuckleDriver ==
  in : Inport
  out : Outport
  wires:
  in/1 -> out/1

== system test_mdl_NI/CAN_Signal/GWM/RCM/RCMStatusMessage2_FD1_4C/ThirdRowBuckleMid ==
  in : Inport
  out : Outport
  wires:
  in/1 -> out/1

== system test_mdl_NI/CAN_Signal/GWM/RCM/RCMStatusMessage2_FD1_4C/ThirdRowBucklePsngr ==
  in : Inport
  out : Outport
  wires:
  in/1 -> out/1

== system test_mdl_NI/CAN_Signal/GWM/SCCM/Steering_Data_FD1_83/AccButtnGapDecPress ==
  in : Inport
  out : Outport
  wires:
  in/1 -> out/1

== system test_mdl_NI/CAN_Signal/GWM/SCCM/Steering_Data_FD1_83/AccButtnGapIncPress ==
  in : Inport
  out : Outport
  wires:
  in/1 -> out/1

== system test_mdl_NI/CAN_Signal/GWM/SCCM/Steering_Data_FD1_83/AccButtnGapTogglePress ==
  in : Inport
  out : Outport
  wires:
  in/1 -> out/1

== system test_mdl_NI/CAN_Signal/GWM/SCCM/Steering_Data_FD1_83/AhbStat_B_Dsply ==
  in : Inport
  out : Outport
  wires:
  in/1 -> out/1

== system test_mdl_NI/CAN_Signal/GWM/SCCM/Steering_Data_FD1_83/AslButtnOnOffCnclPress ==
  in : Inport
  out : Outport
  wires:
  in/1 -> out/1

== system test_mdl_NI/CAN_Signal/GWM/SCCM/Steering_Data_FD1_83/AslButtnOnOffPress ==
  in : Inport
  out : Outport
  wires:
  in/1 -> out/1

== system test_mdl_NI/CAN_Signal/GWM/SCCM/Steering_Data_FD1_83/CcAslButtnCnclPress ==
  in : Inport
  out : Outport
  wires:
  in/1 -> out/1

== system test_mdl_NI/CAN_Signal/GWM/SCCM/Steering_Data_FD1_83/CcAslButtnCnclResPress ==
  in : Inport
  out : Outport
  wires:
  in/1 -> out/1

== system test_mdl_NI/CAN_Signal/GWM/SCCM/Steering_Data_FD1_83/CcAslButtnDeny_B_Actl ==
  in : Inport
  out : Outport
  wires:
  in/1 -> out/1

== system test_mdl_NI/CAN_Signal/GWM/SCCM/Steering_Data_FD1_83/CcAslButtnIndxDecPress ==
  in : Inport
  out : Outport
  wires:
  in/1 -> out/1

== system test_mdl_NI/CAN_Signal/GWM/SCCM/Steering_Data_FD1_83/CcAslButtnIndxIncPress ==
  in : Inport
  out : Outport
  wires:
  in/1 -> out/1

== system test_mdl_NI/CAN_Signal/GWM/SCCM/Steering_Data_FD1_83/CcAslButtnOffCnclPress ==
  in : Inport
  out : Outport
  wires:
  in/1 -> out/1

== system test_mdl_NI/CAN_Signal/GWM/SCCM/Steering_Data_FD1_83/CcAslButtnOnOffCncl ==
  in : Inport
  out : Outport
  wires:
  in/1 -> out/1

== system test_mdl_NI/CAN_Signal/GWM/SCCM/Steering_Data_FD1_83/CcAslButtnOnPress ==
  in : Inport
  out : Outport
  wires:
  in/1 -> out/1

== system test_mdl_NI/CAN_Signal/GWM/SCCM/Steering_Data_FD1_83/CcAslButtnResDecPress ==
  in : Inport
  out : Outport
  wires:
  in/1 -> out/1

== system test_mdl_NI/CAN_Signal/GWM/SCCM/Steering_Data_FD1_83/CcAslButtnResIncPress ==
  in : Inport
  out : Outport
  wires:
  in/1 -> out/1

== system test_mdl_NI/CAN_Signal/GWM/SCCM/Steering_Data_FD1_83/CcAslButtnSetDecPress ==
  in : Inport
  out : Outport
  wires:
  in/1 -> out/1

== system test_mdl_NI/CAN_Signal/GWM/SCCM/Steering_Data_FD1_83/CcAslButtnSetIncPress ==
  in : Inport
  out : Outport
  wires:
  in/1 -> out/1

== system test_mdl_NI/CAN_Signal/GWM/SCCM/Steering_Data_FD1_83/CcAslButtnSetPress ==
  in : Inport
  out : Outport
  wires:
  in/1 -> out/1

== system test_mdl_NI/CAN_Signal/GWM/SCCM/Steering_Data_FD1_83/CcAsllButtnResPress ==
  in : Inport
  out : Outport
  wires:
  in/1 -> out/1

== system test_mdl_NI/CAN_Signal/GWM/SCCM/Steering_Data_FD1_83/CcButtnOffPress ==
  in : Inport
  out : Outport
  wires:
  in/1 -> out/1

== system test_mdl_NI/CAN_Signal/GWM/SCCM/Steering_Data_FD1_83/CcButtnOnOffCnclPress ==
  in : Inport
  out : Outport
  wires:
  in/1 -> out/1

== system test_mdl_NI/CAN_Signal/GWM/SCCM/Steering_Data_FD1_83/CcButtnOnOffPress ==
  in : Inport
  out : Outport
  wires:
  in/1 -> out/1

== system test_mdl_NI/CAN_Signal/GWM/SCCM/Steering_Data_FD1_83/CcButtnOnPress ==
  in : Inport
  out : Outport
  wires:
  in/1 -> out/1

== system test_mdl_NI/CAN_Signal/GWM/SCCM/Steering_Data_FD1_83/HeadLghtHiCtrl_D_RqAhb ==
  in : Inport
  out : Outport
  wires:
  in/1 -> out/1

== system test_mdl_NI/CAN_Signal/GWM/SCCM/Steering_Data_FD1_83/HeadLghtHiFlash_D_Actl ==
  in : Inport
  out : Outport
  wires:
  in/1 -> out/1

== system test_mdl_NI/CAN_Signal/GWM/SCCM/Steering_Data_FD1_83/HeadLghtHiFlash_D_Stat ==
  in : Inport
  out : Outport
  wires:
  in/1 -> out/1

== system test_mdl_NI/CAN_Signal/GWM/SCCM/Steering_Data_FD1_83/HeadLghtHiOn_B_StatAhb ==
  in : Inport
  out : Outport
  wires:
  in/1 -> out/1

== system test_mdl_NI/CAN_Signal/GWM/SCCM/Steering_Data_FD1_83/LaSwtchPos_D_Stat ==
  in : Inport
  out : Outport
  wires:
  in/1 -> out/1

== system test_mdl_NI/CAN_Signal/GWM/SCCM/Steering_Data_FD1_83/LghtAmb_D_Sns ==
  in : Inport
  out : Outport
  wires:
  in/1 -> out/1

== system test_mdl_NI/CAN_Signal/GWM/SCCM/Steering_Data_FD1_83/TjaButtnOnOffPress ==
  in : Inport
  out : Outport
  wires:
  in/1 -> out/1

== system test_mdl_NI/CAN_Signal/GWM/SCCM/Steering_Data_FD1_83/TurnLghtSwtch_D_Stat ==
  in : Inport
  out : Outport
  wires:
  in/1 -> out/1

== system test_mdl_NI/CAN_Signal/GWM/SCCM/Steering_Data_FD1_83/WiprFrontSwtch_D_Stat ==
  in : Inport
  out : Outport
  wires:
  in/1 -> out/1

== system test_mdl_NI/CAN_Signal/GWM/SCCM/Steering_Data_FD1_83/WiprFront_D_Stat ==
  in : Inport
  out : Outport
  wires:
  in/1 -> out/1

== system test_mdl_NI/CAN_Signal/GWM/SCCM/Steering_Wheel_Data2_FD1_81/SelDrvMdeDec_B_RqDrv ==
  in : Inport
  out : Outport
  wires:
  in/1 -> out/1

== system test_mdl_NI/CAN_Signal/GWM/SCCM/Steering_Wheel_Data2_FD1_81/SelDrvMdeInc_B_RqDrv ==
  in : Inport
  out : Outport
  wires:
  in/1 -> out/1

== system test_mdl_NI/CAN_Signal/GWM/SCCM/Steering_Wheel_Data2_FD1_81/SelDrvMdeSwtch_D_Stat4 ==
  in : Inport
  out : Outport
  wires:
  in/1 -> out/1

== system test_mdl_NI/CAN_Signal/GWM/SCCM/Steering_Wheel_Data2_FD1_81/SteEffortInc_B_RqDrv ==
  in : Inport
  out : Outport
  wires:
  in/1 -> out/1

== system test_mdl_NI/CAN_Signal/GWM/SCCM/Steering_Wheel_Data2_FD1_81/SteWhlSwtchBack_B_Stat ==
  in : Inport
  out : Outport
  wires:
  in/1 -> out/1

== system test_mdl_NI/CAN_Signal/GWM/SCCM/Steering_Wheel_Data2_FD1_81/SteWhlSwtchDown_B_Stat ==
  in : Inport
  out : Outport
  wires:
  in/1 -> out/1

== system test_mdl_NI/CAN_Signal/GWM/SCCM/Steering_Wheel_Data2_FD1_81/SteWhlSwtchHome_B_Stat ==
  in : Inport
  out : Outport
  wires:
  in/1 -> out/1

== system test_mdl_NI/CAN_Signal/GWM/SCCM/Steering_Wheel_Data2_FD1_81/SteWhlSwtchHud_B_Stat ==
  in : Inport
  out : Outport
  wires:
  in/1 -> out/1

== system test_mdl_NI/CAN_Signal/GWM/SCCM/Steering_Wheel_Data2_FD1_81/SteWhlSwtchInfo_B_Stat ==
  in : Inport
  out : Outport
  wires:
  in/1 -> out/1

== system test_mdl_NI/CAN_Signal/GWM/SCCM/Steering_Wheel_Data2_FD1_81/SteWhlSwtchIod_B_Stat ==
  in : Inport
  out : Outport
  wires:
  in/1 -> out/1

== system test_mdl_NI/CAN_Signal/GWM/SCCM/Steering_Wheel_Data2_FD1_81/SteWhlSwtchLeft_B_Stat ==
  in : Inport
  out : Outport
  wires:
  in/1 -> out/1

== system test_mdl_NI/CAN_Signal/GWM/SCCM/Steering_Wheel_Data2_FD1_81/SteWhlSwtchMed_B_Stat ==
  in : Inport
  out : Outport
  wires:
  in/1 -> out/1

== system test_mdl_NI/CAN_Signal/GWM/SCCM/Steering_Wheel_Data2_FD1_81/SteWhlSwtchMenu_B_Stat ==
  in : Inport
  out : Outport
  wires:
  in/1 -> out/1

== system test_mdl_NI/CAN_Signal/GWM/SCCM/Steering_Wheel_Data2_FD1_81/SteWhlSwtchNav_B_Stat ==
  in : Inport
  out : Outport
  wires:
  in/1 -> out/1

== system test_mdl_NI/CAN_Signal/GWM/SCCM/Steering_Wheel_Data2_FD1_81/SteWhlSwtchOk_B_Stat ==
  in : Inport
  out : Outport
  wires:
  in/1 -> out/1

== system test_mdl_NI/CAN_Signal/GWM/SCCM/Steering_Wheel_Data2_FD1_81/SteWhlSwtchPhon_B_Stat ==
  in : Inport
  out : Outport
  wires:
  in/1 -> out/1

== system test_mdl_NI/CAN_Signal/GWM/SCCM/Steering_Wheel_Data2_FD1_81/SteWhlSwtchRght_B_Stat ==
  in : Inport
  out : Outport
  wires:
  in/1 -> out/1

== system test_mdl_NI/CAN_Signal/GWM/SCCM/Steering_Wheel_Data2_FD1_81/SteWhlSwtchSet_B_Stat ==
  in : Inport
  out : Outport
  wires:
  in/1 -> out/1

== system test_mdl_NI/CAN_Signal/GWM/SCCM/Steering_Wheel_Data2_FD1_81/SteWhlSwtchUp_B_Stat ==
  in : Inport
  out : Outport
  wires:
  in/1 -> out/1

== system test_mdl_NI/CAN_Signal/GWM/SCCM/Steering_Wheel_Data2_FD1_81/SteWhlSwtchView_B_Stat ==
  in : Inport
  out : Outport
  wires:
  in/1 -> out/1

== system test_mdl_NI/CAN_Signal/GWM/SCCM/Steering_Wheel_Data2_FD1_81/SuspDampInc_B_RqDrv ==
  in : Inport
  out : Outport
  wires:
  in/1 -> out/1

== system test_mdl_NI/CAN_Signal/GWM/Tester_AutoSar/GWM_AutoSar_NetMgmt_FD1/GWM_AutoSarNMControl ==
  in : Inport
  out : Outport
  wires:
  in/1 -> out/1

== system test_mdl_NI/CAN_Signal/GWM/Tester_AutoSar/GWM_AutoSar_NetMgmt_FD1/GWM_AutoSarNMNodeId ==
  in : Inport
  out : Outport
  wires:
  in/1 -> out/1

== system test_mdl_NI/CAN_Signal/GWM/Tester_AutoSar/GWM_AutoSar_NetMgmt_FD1/GWM_AutoSarNMReserved1 ==
  in : Inport
  out : Outport
  wires:
  in/1 -> out/1

== system test_mdl_NI/CAN_Signal/GWM/Tester_AutoSar/GWM_AutoSar_NetMgmt_FD1/GWM_AutoSarNMReserved2 ==
  in : Inport
  out : Outport
  wires:
  in/1 -> out/1

== system test_mdl_NI/CAN_Signal/GWM/Tester_AutoSar/GWM_AutoSar_NetMgmt_FD1/GWM_AutoSarNMReserved3 ==
  in : Inport
  out : Outport
  wires:
  in/1 -> out/1

== system test_mdl_NI/CAN_Signal/GWM/Tester_AutoSar/GWM_AutoSar_NetMgmt_FD1/GWM_AutoSarNMReserved4 ==
  in : Inport
  out : Outport
  wires:
  in/1 -> out/1

== system test_mdl_NI/CAN_Signal/GWM/Tester_AutoSar/GWM_AutoSar_NetMgmt_FD1/GWM_GWNMProxy ==
  in : Inport
  out : Outport
  wires:
  in/1 -> out/1

== system test_mdl_NI/CAN_Signal/GWM/Tester_AutoSar/GWM_AutoSar_NetMgmt_FD1/GWM_GWOnBoardTester ==
  in : Inport
  out : Outport
  wires:
  in/1 -> out/1

== system test_mdl_NI/CAN_Signal/GWM/Tester_AutoSar/TesterPhysicalResGWM_FD1/TesterPhysicalResGWM_F1 ==
  in : Inport
  out : Outport
  wires:
  in/1 -> out/1

== system test_mdl_NI/To_NI_HIL/SRR_L/FL_SOD/SRR_FL_001/SRR_FL_CAN_DET_AMPLITUDE_01 ==
  in : Inport
  out : Outport
  wires:
  in/1 -> out/1

== system test_mdl_NI/To_NI_HIL/SRR_L/FL_SOD/SRR_FL_001/SRR_FL_CAN_DET_AZIMUTH_01 ==
  in : Inport
  out : Outport
  wires:
  in/1 -> out/1

== system test_mdl_NI/To_NI_HIL/SRR_L/FL_SOD/SRR_FL_001/SRR_FL_CAN_DET_ELEVATION_01 ==
  in : Inport
  out : Outport
  wires:
  in/1 -> out/1

== system test_mdl_NI/To_NI_HIL/SRR_L/FL_SOD/SRR_FL_001/SRR_FL_CAN_DET_RANGE_01 ==
  in : Inport
  out : Outport
  wires:
  in/1 -> out/1

== system test_mdl_NI/To_NI_HIL/SRR_L/FL_SOD/SRR_FL_001/SRR_FL_CAN_DET_RANGE_RATE_01 ==
  in : Inport
  out : Outport
  wires:
  in/1 -> out/1

== system test_mdl_NI/To_NI_HIL/SRR_L/FL_SOD/SRR_FL_001/SRR_FL_CAN_DET_SUPER_RES_TARGET_01 ==
  in : Inport
  out : Outport
  wires:
  in/1 -> out/1

== system test_mdl_NI/To_NI_HIL/SRR_L/FL_SOD/SRR_FL_001/SRR_FL_CAN_DET_VALID_LEVEL_01 ==
  in : Inport
  out : Outport
  wires:
  in/1 -> out/1

== system test_mdl_NI/To_NI_HIL/SRR_L/FL_SOD/SRR_FL_002/SRR_FL_CAN_DET_AMPLITUDE_02 ==
  in : Inport
  out : Outport
  wires:
  in/1 -> out/1

== system test_mdl_NI/To_NI_HIL/SRR_L/FL_SOD/SRR_FL_002/SRR_FL_CAN_DET_AZIMUTH_02 ==
  in : Inport
  out : Outport
  wires:
  in/1 -> out/1

== system test_mdl_NI/To_NI_HIL/SRR_L/FL_SOD/SRR_FL_002/SRR_FL_CAN_DET_ELEVATION_02 ==
  in : Inport
  out : Outport
  wires:
  in/1 -> out/1

== system test_mdl_NI/To_NI_HIL/SRR_L/FL_SOD/SRR_FL_002/SRR_FL_CAN_DET_RANGE_02 ==
  in : Inport
  out : Outport
  wires:
  in/1 -> out/1

== system test_mdl_NI/To_NI_HIL/SRR_L/FL_SOD/SRR_FL_002/SRR_FL_CAN_DET_RANGE_RATE_02 ==
  in : Inport
  out : Outport
  wires:
  in/1 -> out/1

== system test_mdl_NI/To_NI_HIL/SRR_L/FL_SOD/SRR_FL_002/SRR_FL_CAN_DET_SUPER_RES_TARGET_02 ==
  in : Inport
  out : Outport
  wires:
  in/1 -> out/1

== system test_mdl_NI/To_NI_HIL/SRR_L/FL_SOD/SRR_FL_002/SRR_FL_CAN_DET_VALID_LEVEL_02 ==
  in : Inport
  out : Outport
  wires:
  in/1 -> out/1

== system test_mdl_NI/To_NI_HIL/SRR_L/FL_SOD/SRR_FL_003/SRR_FL_CAN_DET_AMPLITUDE_03 ==
  in : Inport
  out : Outport
  wires:
  in/1 -> out/1

== system test_mdl_NI/To_NI_HIL/SRR_L/FL_SOD/SRR_FL_003/SRR_FL_CAN_DET_AZIMUTH_03 ==
  in : Inport
  out : Outport
  wires:
  in/1 -> out/1

== system test_mdl_NI/To_NI_HIL/SRR_L/FL_SOD/SRR_FL_003/SRR_FL_CAN_DET_ELEVATION_03 ==
  in : Inport
  out : Outport
  wires:
  in/1 -> out/1

== system test_mdl_NI/To_NI_HIL/SRR_L/FL_SOD/SRR_FL_003/SRR_FL_CAN_DET_RANGE_03 ==
  in : Inport
  out : Outport
  wires:
  in/1 -> out/1

== system test_mdl_NI/To_NI_HIL/SRR_L/FL_SOD/SRR_FL_003/SRR_FL_CAN_DET_RANGE_RATE_03 ==
  in : Inport
  out : Outport
  wires:
  in/1 -> out/1

== system test_mdl_NI/To_NI_HIL/SRR_L/FL_SOD/SRR_FL_003/SRR_FL_CAN_DET_SUPER_RES_TARGET_03 ==
  in : Inport
  out : Outport
  wires:
  in/1 -> out/1

== system test_mdl_NI/To_NI_HIL/SRR_L/FL_SOD/SRR_FL_003/SRR_FL_CAN_DET_VALID_LEVEL_03 ==
  in : Inport
  out : Outport
  wires:
  in/1 -> out/1

== system test_mdl_NI/To_NI_HIL/SRR_L/RL_SOD/SRR_RL_001/SRR_RL_CAN_DET_AMPLITUDE_01 ==
  in : Inport
  out : Outport
  wires:
  in/1 -> out/1

== system test_mdl_NI/To_NI_HIL/SRR_L/RL_SOD/SRR_RL_001/SRR_RL_CAN_DET_AZIMUTH_01 ==
  in : Inport
  out : Outport
  wires:
  in/1 -> out/1

== system test_mdl_NI/To_NI_HIL/SRR_L/RL_SOD/SRR_RL_001/SRR_RL_CAN_DET_ELEVATION_01 ==
  in : Inport
  out : Outport
  wires:
  in/1 -> out/1

== system test_mdl_NI/To_NI_HIL/SRR_L/RL_SOD/SRR_RL_001/SRR_RL_CAN_DET_RANGE_01 ==
  in : Inport
  out : Outport
  wires:
  in/1 -> out/1

== system test_mdl_NI/To_NI_HIL/SRR_L/RL_SOD/SRR_RL_001/SRR_RL_CAN_DET_RANGE_RATE_01 ==
  in : Inport
  out : Outport
  wires:
  in/1 -> out/1

== system test_mdl_NI/To_NI_HIL/SRR_L/RL_SOD/SRR_RL_001/SRR_RL_CAN_DET_SUPER_RES_TARGET_01 ==
  in : Inport
  out : Outport
  wires:
  in/1 -> out/1

== system test_mdl_NI/To_NI_HIL/SRR_L/RL_SOD/SRR_RL_001/SRR_RL_CAN_DET_VALID_LEVEL_01 ==
  in : Inport
  out : Outport
  wires:
  in/1 -> out/1

== system test_mdl_NI/To_NI_HIL/SRR_L/RL_SOD/SRR_RL_002/SRR_RL_CAN_DET_AMPLITUDE_02 ==
  in : Inport
  out : Outport
  wires:
  in/1 -> out/1

== system test_mdl_NI/To_NI_HIL/SRR_L/RL_SOD/SRR_RL_002/SRR_RL_CAN_DET_AZIMUTH_02 ==
  in : Inport
  out : Outport
  wires:
  in/1 -> out/1

== system test_mdl_NI/To_NI_HIL/SRR_L/RL_SOD/SRR_RL_002/SRR_RL_CAN_DET_ELEVATION_02 ==
  in : Inport
  out : Outport
  wires:
  in/1 -> out/1
